simulink model "timeCheck"  (Simulink 8.6)
settings: Solver=VariableStepAuto  StartTime=0.0  StopTime=inf  RelTol=1e-3
settings Model: Creator=Oscar  LastModifiedBy=Oscar
settings DataIOCC: SaveFormat=Dataset  SignalLoggingSaveFormat=Dataset
settings OptimizationCC: ExpressionDepthLimit=128
settings DebuggingCC: UnderspecifiedInitializationDetection=Simplified  MergeDetectMultiDrivingBlocksExec=error  SolverPrmCheckMsg=none  FcnCallInpInsideContextMsg=EnableAllAsError  StateNameClashWarn=none
settings HardwareCC: ProdBitPerPointer=64  ProdLargestAtomicFloat=Float  ProdIntDivRoundTo=Zero  ProdEndianess=LittleEndian  ProdWordSize=64  ProdHWDeviceType=Intel->x86-64 (Windows64)
settings GRTTargetCC: GeneratePreprocessorConditionals=Use local settings  CombineOutputUpdateFcns=on  GRTInterface=off
settings ConfigComp: CovModelRefEnable=off

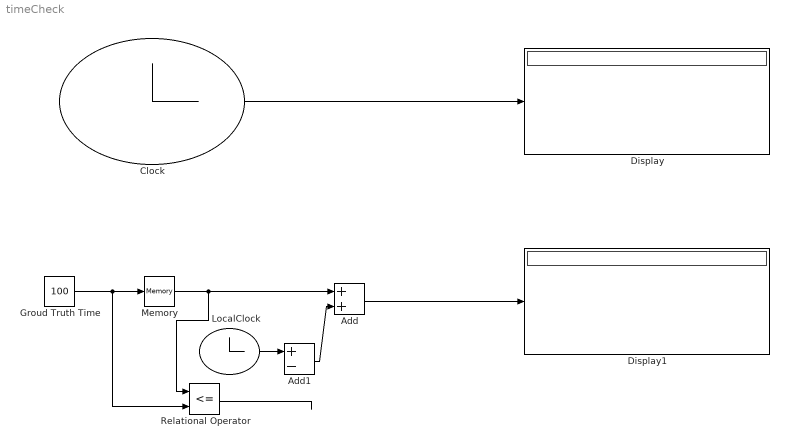
== system timeCheck ==
  Add : Sum
  Add1 : Sum  Inputs=+-
  Clock : Clock
      settings: Decimation=1000
  Display : Display
  Display1 : Display
  Groud Truth Time : Constant  Value=100
  LocalClock : Clock
      settings: Decimation=1000
  Memory : Memory
  Relational Operator : RelationalOperator  Operator=<=  OutDataTypeStr=boolean
  wires:
  Clock/1 -> Display/1
  Groud Truth Time/1 -> Relational Operator/2, Memory/1
  LocalClock/1 -> Add1/1
  Add/1 -> Display1/1
  Memory/1 -> Relational Operator/1, Add/1
  Relational Operator/1 -> ?
  Add1/1 -> Add/2
